simulink model "model_base_bros_old"  (R2017b)
settings: Solver=FixedStepDiscrete  StartTime=0.0  StopTime=inf  FixedStep=sampleTime  RelTol=1e-3
PostLoadFcn:
  | % load model parameters
  | % pname = fileparts(get_param('model_base_bros','filename'));
  | % run([pname  '\parameters_base_model_bros.m']);
  | parameters_base_model_bros;
  | 
  | % set requested state
  | set_param('model_base_bros/Requested state','Value',num2str(0));
InitFcn:
  | % load model parameters
  | % pname = fileparts(get_param('model_base_bros','filename'));
  | % run([pname  '\parameters_base_model_bros.m']);
  | parameters_base_model_bros;
  | 
  | % set requested state
  | set_param('model_base_bros/Requested state','Value',num2str(0));
StartFcn:
  | % load model parameters
  | % pname = fileparts(get_param('model_base_bros','filename'));
  | % run([pname  '\parameters_base_model_bros.m']);
  | parameters_base_model_bros;
  | 
  | % set requested state
  | set_param('model_base_bros/Requested state','Value',num2str(0));
StopFcn:
  | % switch off data logger (to hopefully avoid corrupt files). TwinCAT doesn't properly switch off the logger when shutting down the model
  | % no idea if this'll work.
  | set_param('model_base_bros/Record data (1 = yes, 0 = no)','Value',num2str(0));
values from neighbouring files (symbols this model uses):
  Ax = [0.875562973461 0.676732451464 0.46708754738 0.231474252169]    [data_target_signal.mat]    (also in data_target_signal2.mat = [0.0300392118262 0.0232176440477 0.016025051541 0.0079415236; data_target_signal6.mat = [0.0248342256417 0.0238582232887 0.0214496871858 0.017479383)
  Ay = [0.837910948193 0.637556185526 0.438769549178 0.219632627408]    [data_target_signal.mat]    (also in data_target_signal2.mat = [0.0287474290567 0.0218735669376 0.0150535048079 0.007535255; data_target_signal6.mat = [0.0238582232887 0.022710665482 0.0201288554377 0.0162123456)
  FFMatrix = -[0 -12; 12 0]    [parameters_base_model_bros.m]
  Lb = 0.07    [base_1fm_parameters.m]    (also in parameters_base_model_bros.m)
  Lf = 0.238    [base_1fm_parameters.m]    (also in parameters_base_model_bros.m)
  Lu = 0.153    [base_1fm_parameters.m]    (also in parameters_base_model_bros.m)
  nx = [6 11 17 29]    [data_target_signal.mat]    (also in data_target_signal2.mat; data_target_signal6.mat = [3 4 6 9])
  ny = [7 12 18 30]    [data_target_signal.mat]    (also in data_target_signal2.mat; data_target_signal6.mat = [4 5 7 10])
  phx = [10.4473350794 0.47695350944 4.82715351803 -0.0529087815534]    [data_target_signal.mat]    (also in data_target_signal2.mat = [6.00930363593 0.114916961734 -3.13208164486 9.28056686525]; data_target_signal6.mat = [2.42377070757 8.52431280946 1.18332426876 2.41958419832])
  phy = [-8.14327548903 4.57366609146 -5.09702975105 -0.688854143453]    [data_target_signal.mat]    (also in data_target_signal2.mat = [0.875962873279 6.75046973971 -0.797007663484 -14.3442502222; data_target_signal6.mat = [5.81559481549 13.3925583209 -2.67922656623 -1.93021042965])
  sampleTime = 0.001    [base_1fm_parameters.m]    (also in parameters_base_model_bros.m)
undefined symbols (not defined in the file or in its folder): BROS1, BROS2
libraries: simulink x28, LibraryFM x16, VariousBlocksLibrary x7, simulink_extras x1
(part 3 of 3)

== system model_base_bros_old/Robot1/DataFromEtherCAT/FTSensor_K6D27/spikefilter ==
  in : Inport
  Demux : Demux  Outputs=6
  Mux1 : Mux  Inputs=6
  spike filter oeps : Subsystem
  spike filter oeps1 : Subsystem
  spike filter oeps2 : Subsystem
  spike filter oeps3 : Subsystem
  spike filter oeps4 : Subsystem
  spike filter oeps5 : Subsystem
  out : Outport
  wires:
  spike filter oeps1/1(y) -> Mux1/2
  Mux1/1 -> out/1
  in/1 -> Demux/1
  Demux/3 -> spike filter oeps2/1(u)
  spike filter oeps4/1(y) -> Mux1/5
  spike filter oeps/1(y) -> Mux1/1
  Demux/6 -> spike filter oeps5/1(u)
  spike filter oeps5/1(y) -> Mux1/6
  Demux/1 -> spike filter oeps/1(u)
  Demux/2 -> spike filter oeps1/1(u)
  Demux/4 -> spike filter oeps3/1(u)
  Demux/5 -> spike filter oeps4/1(u)
  spike filter oeps2/1(y) -> Mux1/3
  spike filter oeps3/1(y) -> Mux1/4

== system model_base_bros_old/Robot3/Controller_PD/at home/HoldFirstSampleOnEnable ==
  note: These blocks hold the first sample of the input
      | when the block is enabled (through the action port)
  x : Inport
  Enable : EnablePort  StatesWhenEnabling=reset
  Counter Free-Running : simulink/Sources/Counter Free-Running  NumBits=32  tsamp=-1
  Memory1 : Memory
  Signal Conversion : SignalConversion  OverrideOpt=off
  Switch : Switch  Threshold=1
  x0 : Outport
  wires:
  x/1 -> Switch/3
  Counter Free-Running/1 -> Switch/2
  Memory1/1 -> Switch/1
  Switch/1 -> Signal Conversion/1, Memory1/1
  Signal Conversion/1 -> x0/1

== system model_base_bros_old/Robot3/DataFromEtherCAT/Calculate Arrange Joint and Op Space/forward kinematics ==
  JointPosition_rad : Inport  PortDimensions=[2 1]
  JointVelocity_rads : Inport  Port=2  PortDimensions=[2 1]
  JointAcceleration_rads2 : Inport  Port=3  PortDimensions=[2 1]
  Je : MATLAB Function  TreatAsAtomicUnit=on
  Jedot : MATLAB Function  TreatAsAtomicUnit=on
  Product : Product  Multiplication=Matrix(*)
  calculate xddot : MATLAB Function  TreatAsAtomicUnit=on
  forward kinematics : MATLAB Function  TreatAsAtomicUnit=on
  x : Outport
  xdot : Outport  Port=2
  xddot : Outport  Port=3
  J : Outport  Port=4
  Jdot : Outport  Port=5
  wires:
  JointPosition_rad/1 -> forward kinematics/1(q), Jedot/1(q), Je/1(q)
  Je/1(Je) -> calculate xddot/3(J), Product/1, J/1
  JointVelocity_rads/1 -> calculate xddot/2(qdot), Product/2, Jedot/2(qdot)
  Jedot/1(Jedot) -> calculate xddot/4(Jdot), Jdot/1
  Product/1 -> xdot/1
  forward kinematics/1(x) -> x/1
  calculate xddot/1(xddot) -> xddot/1
  JointAcceleration_rads2/1 -> calculate xddot/1(qddot)

== system model_base_bros_old/Robot3/DataFromEtherCAT/Calculate Arrange Joint and Op Space/forward kinematics1 ==
  JointPosition_rad : Inport  PortDimensions=[2 1]
  JointVelocity_rads : Inport  Port=2  PortDimensions=[2 1]
  JointAcceleration_rads2 : Inport  Port=3  PortDimensions=[2 1]
  Je : MATLAB Function  TreatAsAtomicUnit=on
  Jedot : MATLAB Function  TreatAsAtomicUnit=on
  Product : Product  Multiplication=Matrix(*)
  calculate xddot : MATLAB Function  TreatAsAtomicUnit=on
  forward kinematics : MATLAB Function  TreatAsAtomicUnit=on
  x : Outport
  xdot : Outport  Port=2
  xddot : Outport  Port=3
  J : Outport  Port=4
  Jdot : Outport  Port=5
  wires:
  JointPosition_rad/1 -> forward kinematics/1(q), Jedot/1(q), Je/1(q)
  Je/1(Je) -> calculate xddot/3(J), Product/1, J/1
  JointVelocity_rads/1 -> calculate xddot/2(qdot), Product/2, Jedot/2(qdot)
  Jedot/1(Jedot) -> calculate xddot/4(Jdot), Jdot/1
  Product/1 -> xdot/1
  forward kinematics/1(x) -> x/1
  calculate xddot/1(xddot) -> xddot/1
  JointAcceleration_rads2/1 -> calculate xddot/1(qddot)

== system model_base_bros_old/Robot3/DataFromEtherCAT/FTSensor_K6D27/spikefilter ==
  in : Inport
  Demux : Demux  Outputs=6
  Mux1 : Mux  Inputs=6
  spike filter oeps : Subsystem
  spike filter oeps1 : Subsystem
  spike filter oeps2 : Subsystem
  spike filter oeps3 : Subsystem
  spike filter oeps4 : Subsystem
  spike filter oeps5 : Subsystem
  out : Outport
  wires:
  spike filter oeps1/1(y) -> Mux1/2
  Mux1/1 -> out/1
  in/1 -> Demux/1
  Demux/3 -> spike filter oeps2/1(u)
  spike filter oeps4/1(y) -> Mux1/5
  spike filter oeps/1(y) -> Mux1/1
  Demux/6 -> spike filter oeps5/1(u)
  spike filter oeps5/1(y) -> Mux1/6
  Demux/1 -> spike filter oeps/1(u)
  Demux/2 -> spike filter oeps1/1(u)
  Demux/4 -> spike filter oeps3/1(u)
  Demux/5 -> spike filter oeps4/1(u)
  spike filter oeps2/1(y) -> Mux1/3
  spike filter oeps3/1(y) -> Mux1/4

== system model_base_bros_old/Robot1/DataFromEtherCAT/FTSensor_K6D27/spikefilter/spike filter oeps ==
  u : Inport
  'oeps' filter : MATLAB Function  TreatAsAtomicUnit=on
  Memory : Memory
  Terminator : Terminator
  diff threshold spike : Constant  Value=FTSensorStruct.ThresholdDiffForceSensorSpike
  y : Outport
  wires:
  'oeps' filter/2(y) -> y/1, Memory/1
  diff threshold spike/1 -> 'oeps' filter/2(diffthr)
  Memory/1 -> 'oeps' filter/3(u_prev)
  u/1 -> 'oeps' filter/1(u)
  'oeps' filter/1(isSpike) -> Terminator/1

== system model_base_bros_old/Robot1/DataFromEtherCAT/FTSensor_K6D27/spikefilter/spike filter oeps1 ==
  u : Inport
  'oeps' filter : MATLAB Function  TreatAsAtomicUnit=on
  Memory : Memory
  Terminator : Terminator
  diff threshold spike : Constant  Value=FTSensorStruct.ThresholdDiffForceSensorSpike
  y : Outport
  wires:
  'oeps' filter/2(y) -> y/1, Memory/1
  diff threshold spike/1 -> 'oeps' filter/2(diffthr)
  Memory/1 -> 'oeps' filter/3(u_prev)
  u/1 -> 'oeps' filter/1(u)
  'oeps' filter/1(isSpike) -> Terminator/1

== system model_base_bros_old/Robot1/DataFromEtherCAT/FTSensor_K6D27/spikefilter/spike filter oeps2 ==
  u : Inport
  'oeps' filter : MATLAB Function  TreatAsAtomicUnit=on
  Memory : Memory
  Terminator : Terminator
  diff threshold spike : Constant  Value=FTSensorStruct.ThresholdDiffForceSensorSpike
  y : Outport
  wires:
  'oeps' filter/2(y) -> y/1, Memory/1
  diff threshold spike/1 -> 'oeps' filter/2(diffthr)
  Memory/1 -> 'oeps' filter/3(u_prev)
  u/1 -> 'oeps' filter/1(u)
  'oeps' filter/1(isSpike) -> Terminator/1

== system model_base_bros_old/Robot1/DataFromEtherCAT/FTSensor_K6D27/spikefilter/spike filter oeps3 ==
  u : Inport
  'oeps' filter : MATLAB Function  TreatAsAtomicUnit=on
  Memory : Memory
  Terminator : Terminator
  diff threshold spike : Constant  Value=FTSensorStruct.ThresholdDiffForceSensorSpike
  y : Outport
  wires:
  'oeps' filter/2(y) -> y/1, Memory/1
  diff threshold spike/1 -> 'oeps' filter/2(diffthr)
  Memory/1 -> 'oeps' filter/3(u_prev)
  u/1 -> 'oeps' filter/1(u)
  'oeps' filter/1(isSpike) -> Terminator/1

== system model_base_bros_old/Robot1/DataFromEtherCAT/FTSensor_K6D27/spikefilter/spike filter oeps4 ==
  u : Inport
  'oeps' filter : MATLAB Function  TreatAsAtomicUnit=on
  Memory : Memory
  Terminator : Terminator
  diff threshold spike : Constant  Value=FTSensorStruct.ThresholdDiffForceSensorSpike
  y : Outport
  wires:
  'oeps' filter/2(y) -> y/1, Memory/1
  diff threshold spike/1 -> 'oeps' filter/2(diffthr)
  Memory/1 -> 'oeps' filter/3(u_prev)
  u/1 -> 'oeps' filter/1(u)
  'oeps' filter/1(isSpike) -> Terminator/1

== system model_base_bros_old/Robot1/DataFromEtherCAT/FTSensor_K6D27/spikefilter/spike filter oeps5 ==
  u : Inport
  'oeps' filter : MATLAB Function  TreatAsAtomicUnit=on
  Memory : Memory
  Terminator : Terminator
  diff threshold spike : Constant  Value=FTSensorStruct.ThresholdDiffForceSensorSpike
  y : Outport
  wires:
  'oeps' filter/2(y) -> y/1, Memory/1
  diff threshold spike/1 -> 'oeps' filter/2(diffthr)
  Memory/1 -> 'oeps' filter/3(u_prev)
  u/1 -> 'oeps' filter/1(u)
  'oeps' filter/1(isSpike) -> Terminator/1

== system model_base_bros_old/Robot3/DataFromEtherCAT/FTSensor_K6D27/spikefilter/spike filter oeps ==
  u : Inport
  'oeps' filter : MATLAB Function  TreatAsAtomicUnit=on
  Memory : Memory
  Terminator : Terminator
  diff threshold spike : Constant  Value=FTSensorStruct.ThresholdDiffForceSensorSpike
  y : Outport
  wires:
  'oeps' filter/2(y) -> y/1, Memory/1
  diff threshold spike/1 -> 'oeps' filter/2(diffthr)
  Memory/1 -> 'oeps' filter/3(u_prev)
  u/1 -> 'oeps' filter/1(u)
  'oeps' filter/1(isSpike) -> Terminator/1

== system model_base_bros_old/Robot3/DataFromEtherCAT/FTSensor_K6D27/spikefilter/spike filter oeps1 ==
  u : Inport
  'oeps' filter : MATLAB Function  TreatAsAtomicUnit=on
  Memory : Memory
  Terminator : Terminator
  diff threshold spike : Constant  Value=FTSensorStruct.ThresholdDiffForceSensorSpike
  y : Outport
  wires:
  'oeps' filter/2(y) -> y/1, Memory/1
  diff threshold spike/1 -> 'oeps' filter/2(diffthr)
  Memory/1 -> 'oeps' filter/3(u_prev)
  u/1 -> 'oeps' filter/1(u)
  'oeps' filter/1(isSpike) -> Terminator/1

== system model_base_bros_old/Robot3/DataFromEtherCAT/FTSensor_K6D27/spikefilter/spike filter oeps2 ==
  u : Inport
  'oeps' filter : MATLAB Function  TreatAsAtomicUnit=on
  Memory : Memory
  Terminator : Terminator
  diff threshold spike : Constant  Value=FTSensorStruct.ThresholdDiffForceSensorSpike
  y : Outport
  wires:
  'oeps' filter/2(y) -> y/1, Memory/1
  diff threshold spike/1 -> 'oeps' filter/2(diffthr)
  Memory/1 -> 'oeps' filter/3(u_prev)
  u/1 -> 'oeps' filter/1(u)
  'oeps' filter/1(isSpike) -> Terminator/1

== system model_base_bros_old/Robot3/DataFromEtherCAT/FTSensor_K6D27/spikefilter/spike filter oeps3 ==
  u : Inport
  'oeps' filter : MATLAB Function  TreatAsAtomicUnit=on
  Memory : Memory
  Terminator : Terminator
  diff threshold spike : Constant  Value=FTSensorStruct.ThresholdDiffForceSensorSpike
  y : Outport
  wires:
  'oeps' filter/2(y) -> y/1, Memory/1
  diff threshold spike/1 -> 'oeps' filter/2(diffthr)
  Memory/1 -> 'oeps' filter/3(u_prev)
  u/1 -> 'oeps' filter/1(u)
  'oeps' filter/1(isSpike) -> Terminator/1

== system model_base_bros_old/Robot3/DataFromEtherCAT/FTSensor_K6D27/spikefilter/spike filter oeps4 ==
  u : Inport
  'oeps' filter : MATLAB Function  TreatAsAtomicUnit=on
  Memory : Memory
  Terminator : Terminator
  diff threshold spike : Constant  Value=FTSensorStruct.ThresholdDiffForceSensorSpike
  y : Outport
  wires:
  'oeps' filter/2(y) -> y/1, Memory/1
  diff threshold spike/1 -> 'oeps' filter/2(diffthr)
  Memory/1 -> 'oeps' filter/3(u_prev)
  u/1 -> 'oeps' filter/1(u)
  'oeps' filter/1(isSpike) -> Terminator/1

== system model_base_bros_old/Robot3/DataFromEtherCAT/FTSensor_K6D27/spikefilter/spike filter oeps5 ==
  u : Inport
  'oeps' filter : MATLAB Function  TreatAsAtomicUnit=on
  Memory : Memory
  Terminator : Terminator
  diff threshold spike : Constant  Value=FTSensorStruct.ThresholdDiffForceSensorSpike
  y : Outport
  wires:
  'oeps' filter/2(y) -> y/1, Memory/1
  diff threshold spike/1 -> 'oeps' filter/2(diffthr)
  Memory/1 -> 'oeps' filter/3(u_prev)
  u/1 -> 'oeps' filter/1(u)
  'oeps' filter/1(isSpike) -> Terminator/1

== matlab function model_base_bros_old/Experiment & Haptics/CalculateTrialPerformanceMSE/Calc_RMSE_BROS1 ==
  data: error input; RMSE output
function RMSE = RMSE(error)
% calculate the mean-squared error

persistent N; % number of samples, counter
persistent SSE; % sum of squared of error
if isempty(N), N = 0; end
if isempty(SSE), SSE = 0; end

N = N+1; % new datapoint, increase sample counter

SSE = SSE + norm(error)^2;
RMSE = sqrt(SSE / N);

== matlab function model_base_bros_old/Robot1/DataFromEtherCAT/Calculate Arrange Joint and Op Space/Condition number ==
  data: J input; C output
function C = conditioning(J)
%#codegen

C = norm(J)*norm(pinv(J));

== matlab function model_base_bros_old/Robot1/DataFromEtherCAT/Calculate Arrange Joint and Op Space/forward kinematics1/Je ==
  data: q input; Je output size=[2 2]; Lf parameter; Lu parameter; Lb parameter
function Je = Je( q, Lf, Lu, Lb)
%#codegen

% Calculate the Jacobian for this particular device configuration.
% Note that the function func_eq_Je needs to be in the libraries/kinematis_functions folder

% jacobians
Je = func_eq_Je(q(1),q(2),Lf,Lu,Lb);

== matlab function model_base_bros_old/Robot1/DataFromEtherCAT/Calculate Arrange Joint and Op Space/forward kinematics1/Jedot ==
  data: q input; qdot input; Jedot output size=[2 2]; Lf parameter; Lu parameter; Lb parameter
function Jedot = Jedot( q, qdot, Lf, Lu, Lb)
%#codegen

% Calculate the time derivative of the Jacobian for this particular device configuration.
% Note that the function func_eq_Je needs to be in the libraries/kinematis_functions folder


% jacobians
Jedot = func_eq_Jedot(q(1),q(2),qdot(1),qdot(2),Lf,Lu,Lb);

== matlab function model_base_bros_old/Robot1/DataFromEtherCAT/Calculate Arrange Joint and Op Space/forward kinematics1/calculate xddot ==
  data: qddot input; qdot input size=[2 1]; J input; xddot output size=[2 1]; Jdot input
function xddot = calc_xddot(qddot, qdot, J, Jdot)
%#codegen

xddot = J*qddot + Jdot*qdot;

== matlab function model_base_bros_old/Experiment & Haptics/Target position ==
  data: time input; T input; time_rand input; p output; nx parameter; ny parameter; Ax parameter; Ay parameter; phx parameter; phy parameter; v output
function [p, v]  = msin_target (time, T, time_rand, nx, ny, Ax, Ay, phx, phy) 

% prepare frequencies
dw = 2*pi/T; %w0 depends on trial duration
wx = dw*nx;
wy = dw*ny;

% calculate x and y
px = 0;
py = 0;
vx = 0;
vy = 0;

% randomization
% for every multiple of 20, rotate the target signal
nRand = floor(time_rand/20);
if nRand > 5, nRand = 5; end

% add random starting time (semi-randomization)
time = time + mod(time_rand,20.0);

% calculate sum-of-sines
for i = 1:length(wx)
    % position
    px = px + Ax(i)*sin(wx(i)*time+phx(i));
    py = py + Ay(i)*sin(wy(i)*time+phy(i));
    
    % velocity
    vx = vx + Ax(i)*wx(i)*cos(wx(i)*time+phx(i));
    vy = vy + Ay(i)*wy(i)*cos(wy(i)*time+phy(i));
end

p = [px; py];
v = [vx; vy];

% due to the difference in coordiante systems (of human reaching, y
% forward, x to the right; robot: y towards you and x to the left), rotate
% the target such that it is in a human-centered coordinate system.
p = -p;
v = -v;

% rotate target (to make it more random-appearing)
thetaRot = nRand*(2*pi/6);

R = [cos(thetaRot) -sin(thetaRot); sin(thetaRot) cos(thetaRot)];

p = R*p;
v = R*v;              

end

== matlab function model_base_bros_old/Robot1/DataFromEtherCAT/Calculate Arrange Joint and Op Space/forward kinematics/forward kinematics ==
  data: q input; x output size=[2 1]; Lf parameter; Lu parameter; Lb parameter
function x = FK(q, Lf, Lu, Lb)
%#codegen

% Calculate the endpoint position (forward kinematics)
% Note that the function func_eq_FK needs to be in the libraries/kinematis_functions folder


x = func_eq_FK(q(1),q(2),Lf,Lu,Lb);

== matlab function model_base_bros_old/Robot1/DataFromEtherCAT/Calculate Arrange Joint and Op Space/forward kinematics1/forward kinematics ==
  data: q input; x output size=[2 1]; Lf parameter; Lu parameter; Lb parameter
function x = FK(q, Lf, Lu, Lb)
%#codegen

% Calculate the endpoint position (forward kinematics)
% Note that the function func_eq_FK needs to be in the libraries/kinematis_functions folder


x = func_eq_FK(q(1),q(2),Lf,Lu,Lb);

== matlab function model_base_bros_old/Robot1/DataToEtherCAT/FTSensorError/MATLAB Function ==
  data: ForcesTorques input; e output; MaxForcesTorques input
function e = fcn(ForcesTorques, MaxForcesTorques)

% throw error when any of the forces/torques go over a max allowable value
if any(abs(ForcesTorques) > MaxForcesTorques) 
    e = 1;
else
    e = 0;
end

== matlab function model_base_bros_old/Robot1/Controller_PD/PD + nonlin (op space)/invJ1 ==
  data: x input; J input; y output
function y = invJ(x,J)

y = J.'*x;

== matlab function model_base_bros_old/Robot1/DataFromEtherCAT/Calculate Arrange Joint and Op Space/forward kinematics/Je ==
  data: q input; Je output size=[2 2]; Lf parameter; Lu parameter; Lb parameter
function Je = Je( q, Lf, Lu, Lb)
%#codegen

% Calculate the Jacobian for this particular device configuration.
% Note that the function func_eq_Je needs to be in the libraries/kinematis_functions folder

% jacobians
Je = func_eq_Je(q(1),q(2),Lf,Lu,Lb);

== matlab function model_base_bros_old/Robot1/DataFromEtherCAT/Calculate Arrange Joint and Op Space/forward kinematics/Jedot ==
  data: q input; qdot input; Jedot output size=[2 2]; Lf parameter; Lu parameter; Lb parameter
function Jedot = Jedot( q, qdot, Lf, Lu, Lb)
%#codegen

% Calculate the time derivative of the Jacobian for this particular device configuration.
% Note that the function func_eq_Je needs to be in the libraries/kinematis_functions folder


% jacobians
Jedot = func_eq_Jedot(q(1),q(2),qdot(1),qdot(2),Lf,Lu,Lb);

== matlab function model_base_bros_old/Robot1/DataFromEtherCAT/FTSensor_K6D27/CorrectOffset ==
  data: u_in input; u_out output; reset input; corrected output
function [u_out,corrected] = CorrectOffset(u_in,reset)
%#codegen

persistent data_ offset_ counter_ corrected_;
N = 1000;

% initialize
if isempty(data_)
    data_ = zeros(size(u_in,1), N);
    offset_ = zeros(size(u_in));
    counter_ = 1;
    corrected_ = 0;
end

if (counter_ <= N)
    data_(:,counter_) = u_in;
end

counter_ = counter_ + 1;
if reset
    counter_ = 1;
end

% calculate mean
if counter_ == N
    corrected_ = 1;
    offset_ = mean(data_,2);
end

corrected = corrected_;
u_out = u_in - offset_;

== matlab function model_base_bros_old/Robot1/DataFromEtherCAT/Calculate Arrange Joint and Op Space/IK all joints ==
  data: x input; q_all output; Lf parameter; Lu parameter; Lb parameter
function q_all = IK_all(x,Lf,Lu,Lb)
%#codegen

q_all = func_eqs_IK_all(x(1),x(2),Lf,Lu,Lb);

if any(isnan(q_all)) || any(isinf(q_all))
    q_all = zeros(5,1);
end

== matlab function model_base_bros_old/Robot1/DataFromEtherCAT/Calculate Arrange Joint and Op Space/forward kinematics/calculate xddot ==
  data: qddot input; qdot input size=[2 1]; J input; xddot output size=[2 1]; Jdot input
function xddot = calc_xddot(qddot, qdot, J, Jdot)
%#codegen

xddot = J*qddot + Jdot*qdot;

== matlab function model_base_bros_old/Robot1/Controller_PD/PD + nonlin (op space)/nonlinear compensation ==
  data: J input; Jdot input; qdot input; tau output; RobotStruct parameter
function tau = n(J,Jdot,qdot,RobotStruct)
% mass matrix
phat = RobotStruct.DynModParams;

% select parameters
me = phat(3);
Fs1 = phat(4);
Fv1 = phat(5);
Fs2 = phat(6);
Fv2 = phat(7);

% % jacobians
% J = func_eq_Je(q(1),q(2),Lf,Lu,Lb);
% Jdot = func_eq_Jedot(q(1),q(2),qdot(1),qdot(2),Lf,Lu,Lb);

% calculate joint space mass matrix;
p = [me;Fs1;Fv1;Fs2;Fv2];

% psi 
Psi = [(J'*Jdot)*qdot [ssign(qdot(1)) qdot(1); 0 0] [0 0; ssign(qdot(2)) qdot(2)]];

% torque
tau = Psi*p;

function x = ssign(u,b)
%% x = ssign(u,b)
% soft sign
if nargin < 2
    b = 8;
end

x = 2./(1+exp(-b*u))-1;

== matlab function model_base_bros_old/Experiment & Haptics/CalculateTrialPerformanceMSE/Calc_RMSE_BROS2 ==
  data: error input; RMSE output
function RMSE = RMSE(error)
% calculate the mean-squared error

persistent N; % number of samples, counter
persistent SSE; % sum of squared of error
if isempty(N), N = 0; end
if isempty(SSE), SSE = 0; end

N = N+1; % new datapoint, increase sample counter

SSE = SSE + norm(error)^2;
RMSE = sqrt(SSE / N);

== matlab function model_base_bros_old/Robot1/DataToEtherCAT/CreateSingleErrorValue2/ErrorToPower2 ==
  data: u input; e output
function e = errorToPowerOf2(u)

e = (2.^(0:length(u)-1))*u;

== matlab function model_base_bros_old/Robot1/DataToEtherCAT/CreateSingleErrorValue1/ErrorToPower2 ==
  data: u input; e output
function e = errorToPowerOf2(u)

e = (2.^(0:length(u)-1))*u;

== matlab function model_base_bros_old/Robot1/DataFromEtherCAT/FTSensor_K6D27/SensorToOperationalSpace ==
  data: q_all input; Fs input; FTOpSpace output; transmatside input
function FTOpSpace = ForceSensorToOperationalSpace(q_all,Fs,transmatside)
%#codegen
q1 = q_all(1);
q2 = q_all(2);
q4 = q_all(4);
q5 = q_all(5);

% based on which arm the force sensor is connected
switch transmatside
    case 1
        alpha = pi-q2;   
        beta = q1+alpha-pi/2;
        R0 = rotmat(beta);
        R = blkdiag(R0,R0); % transform forces and moments
    case 2
        alpha = -(pi - q4);
        beta = q5+alpha-pi/2;
        R0 = rotmat(beta);
        R = blkdiag(R0,R0); % transform forces and moments
    otherwise
        R = eye(length(Fs));
end

% transform force
FTOpSpace = R*Fs;

function R = rotmat(q)

R = [cos(q) -sin(q) 0;...
      sin(q)  cos(q) 0;...
      0       0      1];

== matlab function model_base_bros_old/Experiment & Haptics/Admittance // Virtual model1/Virtual Model/Virtual model ==
  data: divTs input; x1 output; xdot1 output; xddot1 output; x2 output size=[2 1]; xdot2 output; xddot2 output; M_v input; B_v input; F1 input; F2 input; x0_1 input; x0_2 input; x1_nompos input; x2_nompos input; Kp_s input; Kd_s input; isConnected input; FFMatrix input; doForceField input; constrainY input; x1_prev input size=2; xdot1_prev input size=2; x2_prev input; xdot2_prev input; sampleTime parameter; Fs1 output; Fs2 output
function [x1,xdot1,xddot1,x2,xdot2,xddot2,Fs1,Fs2] = AC(divTs, M_v, B_v, F1, F2, x0_1, x0_2, x1_nompos,x2_nompos,Kp_s,Kd_s,isConnected,FFMatrix,doForceField,constrainY,x1_prev, xdot1_prev, x2_prev, xdot2_prev, sampleTime)



% constants & limits
div_Ts = max(1,divTs);
Ts = sampleTime/div_Ts;
maxRadius = 0.1;
maxVel = 2.0;
maxAcc = 100.0;
maxForceSpring = 50;
b_b = 0.5; % damping on boundary

% persistents
persistent x1_prev_tmp;
persistent x2_prev_tmp;
persistent onBoundary1;
persistent onBoundary2;

if isempty(x1_prev_tmp), x1_prev_tmp = x0_1;
else, x1_prev_tmp = x1_prev; end 

if isempty(x2_prev_tmp), x2_prev_tmp = x0_2;
else, x2_prev_tmp = x2_prev; end 

if isempty(onBoundary1), onBoundary1 = 0; end
if isempty(onBoundary2), onBoundary2 = 0; end

% lower bounds to mass and damping
m_v = max(0.1,M_v); %lower bound M_v
b_v = max(0,B_v);

if length(m_v) == 1
    m_v1 = m_v;
    m_v2 = m_v;
else
    m_v1 = m_v(1);
    m_v2 = m_v(2);
end

if length(b_v) == 1
    b_v1 = b_v;
    b_v2 = b_v;
else
    b_v1 = b_v(1);
    b_v2 = b_v(2);
end

% assign previous values to x1, x2, xdot1 etc
x1 = x1_prev;
x2 = x2_prev;
xdot1 = xdot1_prev;
xdot2 = xdot1_prev;
xddot1 = [0;0];
xddot2 = [0;0];
Fs1 = [0;0];
Fs2 = [0;0];
% perform integration of virtual dynamics
% using semi-implicit Euler integration

for ii = 1:div_Ts
    % calculate acceleration

    % spring force
    Fs1 = Kp_s*(x2_prev - x1_prev) + Kd_s*(xdot2_prev - xdot1_prev);
    Fs1 = limit(Fs1,maxForceSpring);
    Fs2 = Kp_s*(x1_prev - x2_prev) + Kd_s*(xdot1_prev - xdot2_prev);
    Fs2 = limit(Fs2,maxForceSpring);
    
    if constrainY
        Fs1(2) = 0; 
        Fs2(2) = 0;
    end
    
    % force field
    
    % BROS 1
    xddot1 = (F1 + isConnected*Fs1 + doForceField*FFMatrix*xdot1_prev - b_v1*xdot1_prev - onBoundary1*b_b*xdot1_prev)/m_v1;
    xddot1 = limit(xddot1,maxAcc);

    % BROS 2
    xddot2 = (F2 + isConnected*Fs2 + doForceField*FFMatrix*xdot2_prev - b_v2*xdot2_prev - onBoundary2*b_b*xdot2_prev)/m_v2;
    xddot2 = limit(xddot2,maxAcc);
    
    if constrainY
        xddot1(2) = 0; 
        xddot2(2) = 0;
    end

    % acc -> vel
    % BROS 1
    xdot1 = xdot1_prev + xddot1*Ts;
    [xdot1,lim_vel] = limit(xdot1,maxVel);
    if (lim_vel)
        xddot1 = [0;0];
    end

    % BROS 2
    xdot2 = xdot2_prev + xddot2*Ts;
    [xdot2,lim_vel] = limit(xdot2,maxVel);
    if (lim_vel)
        xddot2 = [0;0];
    end
%     xdot2 = [0;0];
    
    if constrainY
        xdot1(2) = 0; 
        xdot2(2) = 0;
    end

    % vel -> pos
    % BROS 1
    x1 = x1_prev_tmp + xdot1*Ts;

    [x1,lim_pos] = limit(x1-x1_nompos,maxRadius);
    if (lim_pos)
        onBoundary1 = 1;
        unitVec = x1/norm(x1);
        xdot1 = xdot1 - dot(unitVec,xdot1)*unitVec;     % remove normal component
        xddot1 = xddot1 - dot(unitVec,xddot1)*unitVec;  % remove normal component 
    else
        onBoundary1 = 0;
    end
    x1 = x1 + x1_nompos;

    % BROS 2
    x2 = x2_prev_tmp + xdot2*Ts;

    [x2,lim_pos] = limit(x2-x2_nompos,maxRadius);
    if (lim_pos)
        onBoundary2 = 1;
        unitVec = x2/norm(x2);
        xdot2 = xdot2 - dot(unitVec,xdot2)*unitVec;     % remove normal component
        xddot2 = xddot2 - dot(unitVec,xddot2)*unitVec;  % remove normal component 
    else
        onBoundary2 = 0;
    end
    x2 = x2 + x2_nompos;
    
    x1_prev_tmp = x1;
    x2_prev_tmp = x2;
    xdot1_prev = xdot1;
    xdot2_prev = xdot2;
end

end

% limit
function [y,lim] = limit(x,maxVal)
    vecLen = norm(x);
    if vecLen > maxVal
        y = x / vecLen * maxVal;
        lim = 1; 
    else
        y = x;
        lim = 0;
    end
end

== matlab function model_base_bros_old/Robot1/DataToEtherCAT/WorkspacePositionGuard/CheckInternalAngles ==
  data: theta input; angleError output
function angleError = checkInternalErrors(theta)
%#codegen


angleError = 0;
if any(theta([2 4]) >= 0.95*pi)
    angleError = 1;
end

== matlab function model_base_bros_old/Robot1/DataToEtherCAT/WorkspacePositionGuard/EndpointPositionGuard ==
  data: correctState input; xe input; error output
function error = fcn(correctState, xe)
%#codegen


error = 0;

% only check workspace boundaries after homing state is done
if ~correctState 
    return; 
end

% x0 = 0;
% y0 = 0.2354;
% a = 0.11;
% b = 0.08;

% workspace (see design document)
x0 = 0;
y0 = 0.25024;
a = 0.1746;
b = 0.13;%0.1048;

% check if endpoint is outside a predefined ellipse
x = xe(1);
y = xe(2);

% workspace is defined as an ellipse
e = (x-x0)^2 / a^2 + (y-y0)^2 / b^2;

% if is larger than 1, the endpoint is outside the workspace
if e > 1
    error = 1;
end

== matlab function model_base_bros_old/Robot1/DataFromEtherCAT/FTSensor_K6D27/spikefilter/spike filter oeps/'oeps' filter ==
  data: isSpike output; u input; diffthr input; y output; u_prev input
function [isSpike,y] = fcn(u,diffthr,u_prev)
du = u-u_prev;
isSpike = 0;
if (abs(du) > diffthr)
    y = u_prev+sign(du)*diffthr;
    isSpike = 1;
else
    y = u;
end

== matlab function model_base_bros_old/Robot1/DataFromEtherCAT/FTSensor_K6D27/spikefilter/spike filter oeps1/'oeps' filter ==
  data: isSpike output; u input; diffthr input; y output; u_prev input
function [isSpike,y] = fcn(u,diffthr,u_prev)
du = u-u_prev;
isSpike = 0;
if (abs(du) > diffthr)
    y = u_prev+sign(du)*diffthr;
    isSpike = 1;
else
    y = u;
end

== matlab function model_base_bros_old/Robot1/DataFromEtherCAT/FTSensor_K6D27/spikefilter/spike filter oeps2/'oeps' filter ==
  data: isSpike output; u input; diffthr input; y output; u_prev input
function [isSpike,y] = fcn(u,diffthr,u_prev)
du = u-u_prev;
isSpike = 0;
if (abs(du) > diffthr)
    y = u_prev+sign(du)*diffthr;
    isSpike = 1;
else
    y = u;
end

== matlab function model_base_bros_old/Robot1/DataFromEtherCAT/FTSensor_K6D27/spikefilter/spike filter oeps3/'oeps' filter ==
  data: isSpike output; u input; diffthr input; y output; u_prev input
function [isSpike,y] = fcn(u,diffthr,u_prev)
du = u-u_prev;
isSpike = 0;
if (abs(du) > diffthr)
    y = u_prev+sign(du)*diffthr;
    isSpike = 1;
else
    y = u;
end

== matlab function model_base_bros_old/Robot1/DataFromEtherCAT/FTSensor_K6D27/spikefilter/spike filter oeps4/'oeps' filter ==
  data: isSpike output; u input; diffthr input; y output; u_prev input
function [isSpike,y] = fcn(u,diffthr,u_prev)
du = u-u_prev;
isSpike = 0;
if (abs(du) > diffthr)
    y = u_prev+sign(du)*diffthr;
    isSpike = 1;
else
    y = u;
end

== matlab function model_base_bros_old/Robot1/DataFromEtherCAT/FTSensor_K6D27/spikefilter/spike filter oeps5/'oeps' filter ==
  data: isSpike output; u input; diffthr input; y output; u_prev input
function [isSpike,y] = fcn(u,diffthr,u_prev)
du = u-u_prev;
isSpike = 0;
if (abs(du) > diffthr)
    y = u_prev+sign(du)*diffthr;
    isSpike = 1;
else
    y = u;
end

== matlab function model_base_bros_old/Robot3/Controller_PD/PD + nonlin (op space)/invJ1 ==
  data: x input; J input; y output
function y = invJ(x,J)

y = J.'*x;

== matlab function model_base_bros_old/Robot3/Controller_PD/PD + nonlin (op space)/nonlinear compensation ==
  data: J input; Jdot input; qdot input; tau output; RobotStruct parameter
function tau = n(J,Jdot,qdot,RobotStruct)
% mass matrix
phat = RobotStruct.DynModParams;

% select parameters
me = phat(3);
Fs1 = phat(4);
Fv1 = phat(5);
Fs2 = phat(6);
Fv2 = phat(7);

% % jacobians
% J = func_eq_Je(q(1),q(2),Lf,Lu,Lb);
% Jdot = func_eq_Jedot(q(1),q(2),qdot(1),qdot(2),Lf,Lu,Lb);

% calculate joint space mass matrix;
p = [me;Fs1;Fv1;Fs2;Fv2];

% psi 
Psi = [(J'*Jdot)*qdot [ssign(qdot(1)) qdot(1); 0 0] [0 0; ssign(qdot(2)) qdot(2)]];

% torque
tau = Psi*p;

function x = ssign(u,b)
%% x = ssign(u,b)
% soft sign
if nargin < 2
    b = 8;
end

x = 2./(1+exp(-b*u))-1;

== matlab function model_base_bros_old/Robot3/DataFromEtherCAT/Calculate Arrange Joint and Op Space/Condition number ==
  data: J input; C output
function C = conditioning(J)
%#codegen

C = norm(J)*norm(pinv(J));

== matlab function model_base_bros_old/Robot3/DataFromEtherCAT/Calculate Arrange Joint and Op Space/IK all joints ==
  data: x input; q_all output; Lf parameter; Lu parameter; Lb parameter
function q_all = IK_all(x,Lf,Lu,Lb)
%#codegen

q_all = func_eqs_IK_all(x(1),x(2),Lf,Lu,Lb);

if any(isnan(q_all)) || any(isinf(q_all))
    q_all = zeros(5,1);
end

== matlab function model_base_bros_old/Robot3/DataFromEtherCAT/Calculate Arrange Joint and Op Space/forward kinematics/Je ==
  data: q input; Je output size=[2 2]; Lf parameter; Lu parameter; Lb parameter
function Je = Je( q, Lf, Lu, Lb)
%#codegen

% Calculate the Jacobian for this particular device configuration.
% Note that the function func_eq_Je needs to be in the libraries/kinematis_functions folder

% jacobians
Je = func_eq_Je(q(1),q(2),Lf,Lu,Lb);

== matlab function model_base_bros_old/Robot3/DataFromEtherCAT/Calculate Arrange Joint and Op Space/forward kinematics/Jedot ==
  data: q input; qdot input; Jedot output size=[2 2]; Lf parameter; Lu parameter; Lb parameter
function Jedot = Jedot( q, qdot, Lf, Lu, Lb)
%#codegen

% Calculate the time derivative of the Jacobian for this particular device configuration.
% Note that the function func_eq_Je needs to be in the libraries/kinematis_functions folder


% jacobians
Jedot = func_eq_Jedot(q(1),q(2),qdot(1),qdot(2),Lf,Lu,Lb);

== matlab function model_base_bros_old/Robot3/DataFromEtherCAT/Calculate Arrange Joint and Op Space/forward kinematics/calculate xddot ==
  data: qddot input; qdot input size=[2 1]; J input; xddot output size=[2 1]; Jdot input
function xddot = calc_xddot(qddot, qdot, J, Jdot)
%#codegen

xddot = J*qddot + Jdot*qdot;

== matlab function model_base_bros_old/Robot3/DataFromEtherCAT/Calculate Arrange Joint and Op Space/forward kinematics/forward kinematics ==
  data: q input; x output size=[2 1]; Lf parameter; Lu parameter; Lb parameter
function x = FK(q, Lf, Lu, Lb)
%#codegen

% Calculate the endpoint position (forward kinematics)
% Note that the function func_eq_FK needs to be in the libraries/kinematis_functions folder


x = func_eq_FK(q(1),q(2),Lf,Lu,Lb);

== matlab function model_base_bros_old/Robot3/DataFromEtherCAT/Calculate Arrange Joint and Op Space/forward kinematics1/Je ==
  data: q input; Je output size=[2 2]; Lf parameter; Lu parameter; Lb parameter
function Je = Je( q, Lf, Lu, Lb)
%#codegen

% Calculate the Jacobian for this particular device configuration.
% Note that the function func_eq_Je needs to be in the libraries/kinematis_functions folder

% jacobians
Je = func_eq_Je(q(1),q(2),Lf,Lu,Lb);

== matlab function model_base_bros_old/Robot3/DataFromEtherCAT/Calculate Arrange Joint and Op Space/forward kinematics1/Jedot ==
  data: q input; qdot input; Jedot output size=[2 2]; Lf parameter; Lu parameter; Lb parameter
function Jedot = Jedot( q, qdot, Lf, Lu, Lb)
%#codegen

% Calculate the time derivative of the Jacobian for this particular device configuration.
% Note that the function func_eq_Je needs to be in the libraries/kinematis_functions folder


% jacobians
Jedot = func_eq_Jedot(q(1),q(2),qdot(1),qdot(2),Lf,Lu,Lb);

== matlab function model_base_bros_old/Robot3/DataFromEtherCAT/Calculate Arrange Joint and Op Space/forward kinematics1/calculate xddot ==
  data: qddot input; qdot input size=[2 1]; J input; xddot output size=[2 1]; Jdot input
function xddot = calc_xddot(qddot, qdot, J, Jdot)
%#codegen

xddot = J*qddot + Jdot*qdot;

== matlab function model_base_bros_old/Robot3/DataFromEtherCAT/Calculate Arrange Joint and Op Space/forward kinematics1/forward kinematics ==
  data: q input; x output size=[2 1]; Lf parameter; Lu parameter; Lb parameter
function x = FK(q, Lf, Lu, Lb)
%#codegen

% Calculate the endpoint position (forward kinematics)
% Note that the function func_eq_FK needs to be in the libraries/kinematis_functions folder


x = func_eq_FK(q(1),q(2),Lf,Lu,Lb);

== matlab function model_base_bros_old/Robot3/DataFromEtherCAT/FTSensor_K6D27/CorrectOffset ==
  data: u_in input; u_out output; reset input; corrected output
function [u_out,corrected] = CorrectOffset(u_in,reset)
%#codegen

persistent data_ offset_ counter_ corrected_;
N = 1000;

% initialize
if isempty(data_)
    data_ = zeros(size(u_in,1), N);
    offset_ = zeros(size(u_in));
    counter_ = 1;
    corrected_ = 0;
end

if (counter_ <= N)
    data_(:,counter_) = u_in;
end

counter_ = counter_ + 1;
if reset
    counter_ = 1;
end

% calculate mean
if counter_ == N
    corrected_ = 1;
    offset_ = mean(data_,2);
end

corrected = corrected_;
u_out = u_in - offset_;

== matlab function model_base_bros_old/Robot3/DataFromEtherCAT/FTSensor_K6D27/SensorToOperationalSpace ==
  data: q_all input; Fs input; FTOpSpace output; transmatside input
function FTOpSpace = ForceSensorToOperationalSpace(q_all,Fs,transmatside)
%#codegen
q1 = q_all(1);
q2 = q_all(2);
q4 = q_all(4);
q5 = q_all(5);

% based on which arm the force sensor is connected
switch transmatside
    case 1
        alpha = pi-q2;   
        beta = q1+alpha-pi/2;
        R0 = rotmat(beta);
        R = blkdiag(R0,R0); % transform forces and moments
    case 2
        alpha = -(pi - q4);
        beta = q5+alpha-pi/2;
        R0 = rotmat(beta);
        R = blkdiag(R0,R0); % transform forces and moments
    otherwise
        R = eye(length(Fs));
end

% transform force
FTOpSpace = R*Fs;

function R = rotmat(q)

R = [cos(q) -sin(q) 0;...
      sin(q)  cos(q) 0;...
      0       0      1];

== matlab function model_base_bros_old/Robot3/DataFromEtherCAT/FTSensor_K6D27/spikefilter/spike filter oeps/'oeps' filter ==
  data: isSpike output; u input; diffthr input; y output; u_prev input
function [isSpike,y] = fcn(u,diffthr,u_prev)
du = u-u_prev;
isSpike = 0;
if (abs(du) > diffthr)
    y = u_prev+sign(du)*diffthr;
    isSpike = 1;
else
    y = u;
end

== matlab function model_base_bros_old/Robot3/DataFromEtherCAT/FTSensor_K6D27/spikefilter/spike filter oeps1/'oeps' filter ==
  data: isSpike output; u input; diffthr input; y output; u_prev input
function [isSpike,y] = fcn(u,diffthr,u_prev)
du = u-u_prev;
isSpike = 0;
if (abs(du) > diffthr)
    y = u_prev+sign(du)*diffthr;
    isSpike = 1;
else
    y = u;
end

== matlab function model_base_bros_old/Robot3/DataFromEtherCAT/FTSensor_K6D27/spikefilter/spike filter oeps2/'oeps' filter ==
  data: isSpike output; u input; diffthr input; y output; u_prev input
function [isSpike,y] = fcn(u,diffthr,u_prev)
du = u-u_prev;
isSpike = 0;
if (abs(du) > diffthr)
    y = u_prev+sign(du)*diffthr;
    isSpike = 1;
else
    y = u;
end

== matlab function model_base_bros_old/Robot3/DataFromEtherCAT/FTSensor_K6D27/spikefilter/spike filter oeps3/'oeps' filter ==
  data: isSpike output; u input; diffthr input; y output; u_prev input
function [isSpike,y] = fcn(u,diffthr,u_prev)
du = u-u_prev;
isSpike = 0;
if (abs(du) > diffthr)
    y = u_prev+sign(du)*diffthr;
    isSpike = 1;
else
    y = u;
end

== matlab function model_base_bros_old/Robot3/DataFromEtherCAT/FTSensor_K6D27/spikefilter/spike filter oeps4/'oeps' filter ==
  data: isSpike output; u input; diffthr input; y output; u_prev input
function [isSpike,y] = fcn(u,diffthr,u_prev)
du = u-u_prev;
isSpike = 0;
if (abs(du) > diffthr)
    y = u_prev+sign(du)*diffthr;
    isSpike = 1;
else
    y = u;
end

== matlab function model_base_bros_old/Robot3/DataFromEtherCAT/FTSensor_K6D27/spikefilter/spike filter oeps5/'oeps' filter ==
  data: isSpike output; u input; diffthr input; y output; u_prev input
function [isSpike,y] = fcn(u,diffthr,u_prev)
du = u-u_prev;
isSpike = 0;
if (abs(du) > diffthr)
    y = u_prev+sign(du)*diffthr;
    isSpike = 1;
else
    y = u;
end

== matlab function model_base_bros_old/Robot3/DataToEtherCAT/CreateSingleErrorValue1/ErrorToPower2 ==
  data: u input; e output
function e = errorToPowerOf2(u)

e = (2.^(0:length(u)-1))*u;

== matlab function model_base_bros_old/Robot3/DataToEtherCAT/CreateSingleErrorValue2/ErrorToPower2 ==
  data: u input; e output
function e = errorToPowerOf2(u)

e = (2.^(0:length(u)-1))*u;

== matlab function model_base_bros_old/Robot3/DataToEtherCAT/FTSensorError/MATLAB Function ==
  data: ForcesTorques input; e output; MaxForcesTorques input
function e = fcn(ForcesTorques, MaxForcesTorques)

% throw error when any of the forces/torques go over a max allowable value
if any(abs(ForcesTorques) > MaxForcesTorques) 
    e = 1;
else
    e = 0;
end

== matlab function model_base_bros_old/Robot3/DataToEtherCAT/WorkspacePositionGuard/CheckInternalAngles ==
  data: theta input; angleError output
function angleError = checkInternalErrors(theta)
%#codegen


angleError = 0;
if any(theta([2 4]) >= 0.95*pi)
    angleError = 1;
end

== matlab function model_base_bros_old/Robot3/DataToEtherCAT/WorkspacePositionGuard/EndpointPositionGuard ==
  data: correctState input; xe input; error output
function error = fcn(correctState, xe)
%#codegen


error = 0;

% only check workspace boundaries after homing state is done
if ~correctState 
    return; 
end

% x0 = 0;
% y0 = 0.2354;
% a = 0.11;
% b = 0.08;

% workspace (see design document)
x0 = 0;
y0 = 0.25024;
a = 0.1746;
b = 0.13;%0.1048;

% check if endpoint is outside a predefined ellipse
x = xe(1);
y = xe(2);

% workspace is defined as an ellipse
e = (x-x0)^2 / a^2 + (y-y0)^2 / b^2;

% if is larger than 1, the endpoint is outside the workspace
if e > 1
    error = 1;
end
